simulink model "Example_DAE"  (R2025b)
settings: Solver=VariableStepAuto  StartTime=0.0  StopTime=10.0  RelTol=1e-3
settings Model: Creator=georg  LastModifiedBy=georg

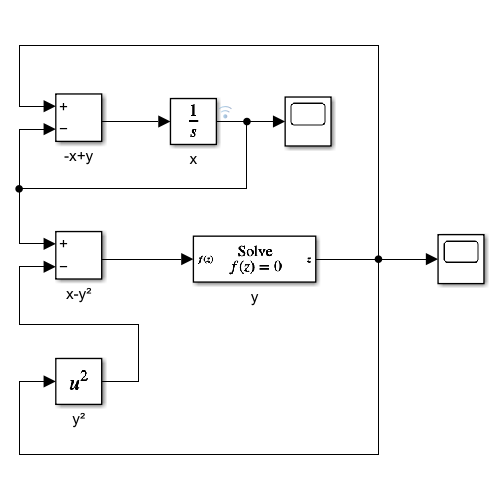
[thumbnail: Simulink's stored preview of the top-level diagram]
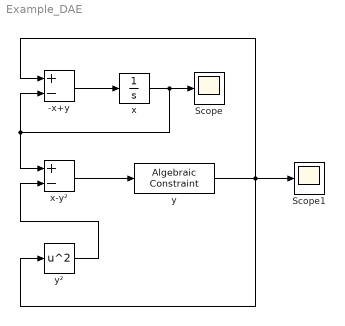
== system Example_DAE ==
  -x+y : Sum  Inputs=+-
  Scope : Scope
      settings: ActiveDisplayYMinimum=-0.091980247076487442  ActiveDisplayYMaximum=11.121331138564054
  Scope1 : Scope
      settings: ActiveDisplayYMinimum=-0.10860952253886769  ActiveDisplayYMaximum=11.123178835837653
  x : Integrator  InitialCondition=10
  x-y² : Sum  Inputs=+-
  y : AlgebraicConstraint
  y² : Math  Operator=square
  wires:
  x/1 -> Scope/1, -x+y/2, x-y²/1
  y/1 -> Scope1/1, y²/1, -x+y/1
  -x+y/1 -> x/1
  x-y²/1 -> y/1
  y²/1 -> x-y²/2
